simulink model "sampleModel1526"  (R2023a)
settings: Solver=VariableStepAuto  StartTime=0.0  StopTime=10.0  RelTol=1e-3
libraries: hdlsllib x2
settings Model: Creator=user1  LastModifiedBy=user1

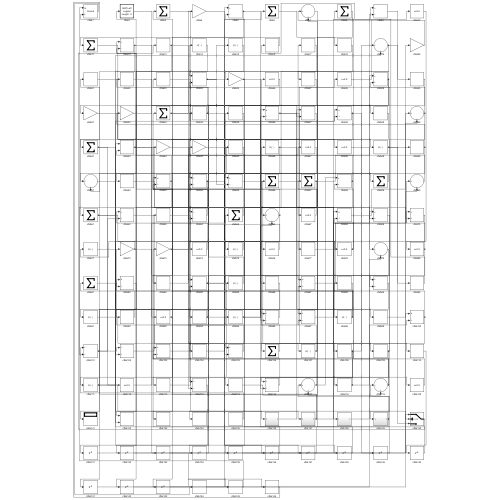
[thumbnail: Simulink's stored preview of the top-level diagram]
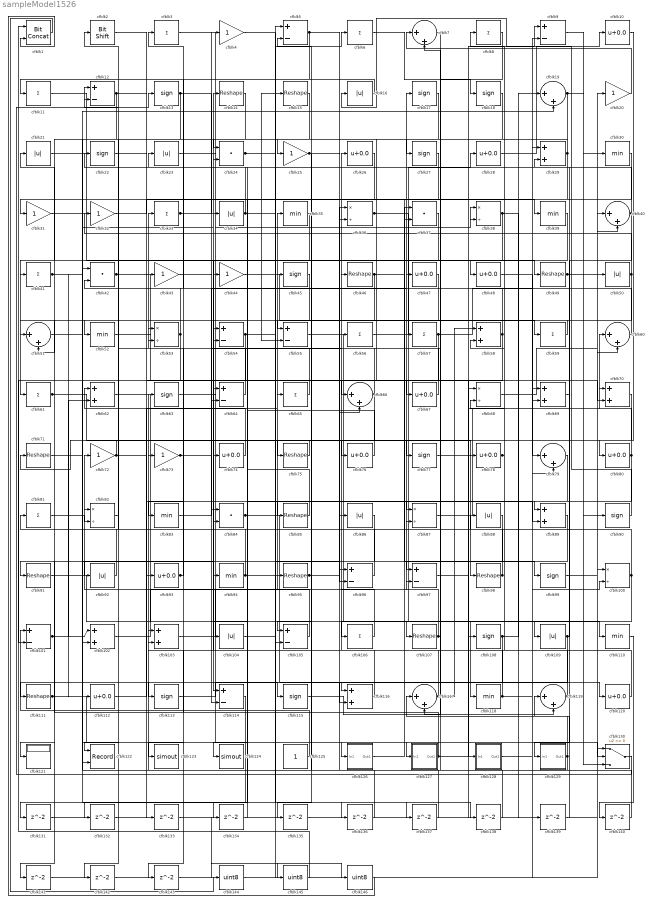
== system sampleModel1526 ==
  cfblk1 : hdlsllib/Logic and Bit Operations/Bit Concat  numInputs=2
  cfblk{10,26,28,47..48,67,74,76,78,80,93,112,120} (13 alike) : Bias  Bias=0.0  SaturateOnIntegerOverflow=off
  cfblk{36,38,53,68,82,87,100} (7 alike) : Product  Inputs=*/  RndMeth=Zero  SaturateOnIntegerOverflow=on
  cfblk{5,9,12,54..55,64,96..97,101,105,114} (11 alike) : Sum  Inputs=+-
  cfblk{29,58,62,69..70,89,102..103,116} (9 alike) : Sum
  cfblk{16,21,23,34,50,86,88,92,104,109} (10 alike) : Abs  SaturateOnIntegerOverflow=off
  cfblk{3,6,8,11,33,41,56..57,59,61,65,81,106} (13 alike) : Sum  Inputs=+
  cfblk{14..15,46,49,71,75,85,91,95,98,107,111} (12 alike) : Reshape
  cfblk{13,17..18,22,27,45,63,77,90,99,108,113,115} (13 alike) : Signum
  cfblk{30,35,39,52,83,94,110,118} (8 alike) : MinMax
  cfblk{7,19,40,51,60,66,79,117,119} (9 alike) : Sum  Inputs=|++
  cfblk121 : Display
  cfblk122 : Record  FileSettingsInternal="{\"entries\":[{\"content\":{\"excelSettings\":{\"content\":{},\"type\":\"Streamout.ExcelSettings\"}},\"type\":\"Streamout.FileSettingStorage\",\"uuid\":\"\"}],\"packageUris\":[\"http:\\/\\/schema.mathworks.com\\/mf0\\/streamout_blocks\\/R2020a\"],\"version\":\"1.0\"}"  Layout=[1 1]  SignalsInternal="{\"entries\":[{\"content\":{},\"type\":\"RecordBlkView.InputSignals\",\"uuid\":\"\"}],\"packageUris\":[\"http:\\/\\/schema.mathworks.com\\/mf0\\/streamout_blocks\\/R2020a\"],\"version\":\"1.0\"}"  VisualizationBindings="{\"xyplotplugin\":{\"info\":[{\"series\":[{\"bindingParametersList\":[{\"parameter\":\"X-Axis\",\"signalID\":1531,\"signalName\":\"cfblk82\"},{\"parameter\":\"Y-Axis\",\"signalID\":1535,\"signalName\":\"cfblk12\"}],\"seriesID\":53253}],\"subplotID\":1}]}}"  CompatibilityTag=XY  st=-1
  cfblk123 : ToWorkspace  VariableName=simout  SaveFormat=Timeseries  SampleTime=-1
  cfblk124 : ToWorkspace  VariableName=simout  SaveFormat=Timeseries  SampleTime=-1
  cfblk125 : Constant  SampleTime=-1
  cfblk126 : Subsystem
      settings: LibrarySourceBlock=|
      | hdlsllib/Ports &
      | Subsystems/Subsystem
  cfblk127 : Subsystem
      settings: LibrarySourceBlock=|
      | hdlsllib/Ports &
      | Subsystems/Subsystem
  cfblk128 : Subsystem
      settings: LibrarySourceBlock=|
      | hdlsllib/Ports &
      | Subsystems/Subsystem
  cfblk129 : Subsystem
      settings: LibrarySourceBlock=|
      | hdlsllib/Ports &
      | Subsystems/Subsystem
  cfblk130 : Switch  SaturateOnIntegerOverflow=off  InputSameDT=off
  cfblk{131..143} (13 alike) : Delay  SampleTime=1
  cfblk144 : DataTypeConversion  OutDataTypeStr=uint8  SaturateOnIntegerOverflow=off  RndMeth=Floor
  cfblk145 : DataTypeConversion  OutDataTypeStr=uint8  SaturateOnIntegerOverflow=off  RndMeth=Floor
  cfblk146 : DataTypeConversion  OutDataTypeStr=uint8  SaturateOnIntegerOverflow=off  RndMeth=Floor
  cfblk2 : hdlsllib/Logic and Bit Operations/Bit Shift  mode=Shift Left Logical  N=0
  cfblk{4,20,25,31..32,43..44,72..73} (9 alike) : Gain
  cfblk{24,37,42,84} (4 alike) : DotProduct  OutDataTypeStr=Inherit: Inherit via internal rule
  wires:
  cfblk3/1 -> cfblk127/1(In1)
  cfblk62/1 -> cfblk107/1
  cfblk113/1 -> cfblk115/1
  cfblk79/1 -> cfblk116/1
  cfblk9/1 -> cfblk30/1
  cfblk23/1 -> cfblk48/1
  cfblk78/1 -> cfblk8/1, cfblk58/2
  cfblk69/1 -> cfblk129/1(In1)
  cfblk129/1(Out1) -> cfblk63/1, cfblk57/1
  cfblk92/1 -> cfblk72/1
  cfblk118/1 -> cfblk26/1, cfblk79/2
  cfblk80/1 -> cfblk60/1, cfblk124/1
  cfblk57/1 -> cfblk114/1, cfblk29/1
  cfblk117/1 -> cfblk73/1, cfblk58/1
  cfblk21/1 -> cfblk114/2
  cfblk116/1 -> cfblk14/1
  cfblk13/1 -> cfblk52/1, cfblk105/2
  cfblk16/1 -> cfblk11/1
  cfblk33/1 -> cfblk4/1, cfblk38/2
  cfblk17/1 -> cfblk25/1
  cfblk64/1 -> cfblk33/1
  cfblk125/1 -> cfblk101/1
  cfblk55/1 -> cfblk110/1
  cfblk75/1 -> cfblk74/1
  cfblk90/1 -> cfblk16/1
  cfblk130/1 -> cfblk13/1
  cfblk20/1 -> cfblk7/1
  cfblk60/1 -> cfblk42/2
  cfblk106/1 -> cfblk46/1
  cfblk18/1 -> cfblk66/1
  cfblk63/1 -> cfblk98/1
  cfblk44/1 -> cfblk59/1
  cfblk88/1 -> cfblk111/1
  cfblk37/1 -> cfblk113/1
  cfblk101/1 -> cfblk102/1, cfblk62/2
  cfblk25/1 -> cfblk87/1, cfblk135/1
  cfblk73/1 -> cfblk84/1, cfblk47/1
  cfblk10/1 -> cfblk80/1
  cfblk74/1 -> cfblk62/1
  cfblk97/1 -> cfblk9/1
  cfblk36/1 -> cfblk118/1, cfblk99/1
  cfblk32/1 -> cfblk39/1
  cfblk107/1 -> cfblk17/1, cfblk87/2
  cfblk83/1 -> cfblk56/1
  cfblk91/1 -> cfblk109/1
  cfblk72/1 -> cfblk71/1, cfblk89/2
  cfblk41/1 -> cfblk94/1, cfblk112/1
  cfblk42/1 -> cfblk108/1, cfblk70/2
  cfblk77/1 -> cfblk9/2
  cfblk45/1 -> cfblk123/1
  cfblk5/1 -> cfblk83/1, cfblk49/1
  cfblk95/1 -> cfblk36/2, cfblk66/2
  cfblk38/1 -> cfblk85/1, cfblk139/1
  cfblk103/1 -> cfblk35/1
  cfblk27/1 -> cfblk31/1
  cfblk52/1 -> cfblk128/1(In1)
  cfblk40/1 -> cfblk89/1, cfblk12/1
  cfblk65/1 -> cfblk43/1
  cfblk35/1 -> cfblk64/1
  cfblk24/1 -> cfblk15/1, cfblk78/1, cfblk55/2
  cfblk28/1 -> cfblk10/1
  cfblk54/1 -> cfblk101/2, cfblk136/1
  cfblk93/1 -> cfblk53/1, cfblk143/1
  cfblk11/1 -> cfblk86/1
  cfblk105/1 -> cfblk82/1
  cfblk99/1 -> cfblk40/1
  cfblk87/1 -> cfblk20/1
  cfblk115/1 -> cfblk119/2
  cfblk82/1 -> cfblk122/1
  cfblk26/1 -> cfblk104/1
  cfblk59/1 -> cfblk55/1
  cfblk127/1(Out1) -> cfblk81/1, cfblk103/2, cfblk70/1
  cfblk22/1 -> cfblk93/1
  cfblk89/1 -> cfblk121/1
  cfblk56/1 -> cfblk28/1
  cfblk112/1 -> cfblk65/1
  cfblk96/1 -> cfblk22/1
  cfblk86/1 -> cfblk91/1
  cfblk12/1 -> cfblk122/2, cfblk37/2
  cfblk94/1 -> cfblk21/1, cfblk6/1
  cfblk48/1 -> cfblk79/1
  cfblk68/1 -> cfblk50/1
  cfblk7/1 -> cfblk97/1
  cfblk109/1 -> cfblk116/2, cfblk29/2
  cfblk81/1 -> cfblk82/2
  cfblk98/1 -> cfblk7/2, cfblk24/2
  cfblk61/1 -> cfblk76/1, cfblk19/2
  cfblk120/1 -> cfblk88/1
  cfblk39/1 -> cfblk61/1
  cfblk49/1 -> cfblk40/2, cfblk90/1
  cfblk14/1 -> cfblk41/1
  cfblk102/1 -> cfblk97/2
  cfblk111/1 -> cfblk126/1(In1), cfblk34/1
  cfblk8/1 -> cfblk67/1
  cfblk47/1 -> cfblk51/1
  cfblk19/1 -> cfblk24/1, cfblk130/3
  cfblk100/1 -> cfblk53/2, cfblk106/1
  cfblk70/1 -> cfblk75/1
  cfblk67/1 -> cfblk45/1
  cfblk58/1 -> cfblk3/1, cfblk105/1
  cfblk76/1 -> cfblk44/1
  cfblk46/1 -> cfblk54/1, cfblk69/2
  cfblk50/1 -> cfblk51/2, cfblk32/1
  cfblk84/1 -> cfblk120/1, cfblk38/1
  cfblk66/1 -> cfblk102/2, cfblk12/2
  cfblk6/1 -> cfblk18/1
  cfblk53/1 -> cfblk2/1, cfblk132/1
  cfblk85/1 -> cfblk54/2
  cfblk31/1 -> cfblk96/1
  cfblk128/1(Out1) -> cfblk100/2
  cfblk43/1 -> cfblk64/2
  cfblk51/1 -> cfblk130/2
  cfblk15/1 -> cfblk92/1
  cfblk126/1(Out1) -> cfblk37/1
  cfblk34/1 -> cfblk23/1, cfblk96/2
  cfblk108/1 -> cfblk117/2, cfblk19/1, cfblk131/1
  cfblk119/1 -> cfblk68/2, cfblk103/1
  cfblk104/1 -> cfblk5/1
  cfblk29/1 -> cfblk77/1, cfblk27/1, cfblk142/1
  cfblk131/1 -> cfblk60/2
  cfblk132/1 -> cfblk100/1
  cfblk2/1 -> cfblk133/1
  cfblk30/1 -> cfblk134/1
  cfblk134/1 -> cfblk84/2
  cfblk135/1 -> cfblk68/1
  cfblk136/1 -> cfblk5/2
  cfblk71/1 -> cfblk137/1
  cfblk137/1 -> cfblk42/1
  cfblk4/1 -> cfblk138/1
  cfblk138/1 -> cfblk117/1
  cfblk139/1 -> cfblk119/1
  cfblk110/1 -> cfblk140/1
  cfblk140/1 -> cfblk36/1
  cfblk114/1 -> cfblk141/1
  cfblk141/1 -> cfblk130/1
  cfblk142/1 -> cfblk69/1
  cfblk1/1 -> cfblk144/1
  cfblk144/1 -> cfblk95/1
  cfblk133/1 -> cfblk145/1
  cfblk145/1 -> cfblk1/1
  cfblk143/1 -> cfblk146/1
  cfblk146/1 -> cfblk1/2

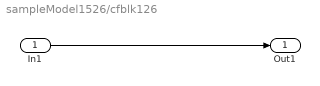
== system sampleModel1526/cfblk126 ==
  In1 : Inport
  Out1 : Outport
  wires:
  In1/1 -> Out1/1

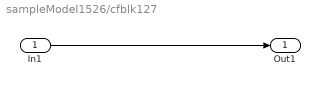
== system sampleModel1526/cfblk127 ==
  In1 : Inport
  Out1 : Outport
  wires:
  In1/1 -> Out1/1

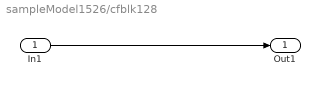
== system sampleModel1526/cfblk128 ==
  In1 : Inport
  Out1 : Outport
  wires:
  In1/1 -> Out1/1

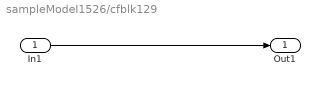
== system sampleModel1526/cfblk129 ==
  In1 : Inport
  Out1 : Outport
  wires:
  In1/1 -> Out1/1
